simulink model "ibvs_lite_model"  (R2020b)
settings: Solver=ode45  StartTime=0.0  StopTime=inf  RelTol=1e-3  EnableMultiTasking=on
values from neighbouring files (symbols this model uses):
  q0 = zeros(7,1)    [setup.m]
  x0 = [T.t', tr2rpy(T)]    [setup.m]
undefined symbols (not defined in the file or in its folder): cond, LWR, mkgrid, nofriction, transl, troty, trotz
libraries: roblocks x19, simulink x4
(part 2 of 2)

== matlab function ibvs_lite_model/inverse_dyn ==
  data: q input; tau output; dq input; ddq input
function tau = idm(q, dq, ddq)

q1 = q(1);
q2 = q(2);
q3 = q(3);
q4 = q(4);
q5 = q(5);
q6 = q(6);
q7 = q(7);

QP1 = dq(1);
QP2 = dq(2);
QP3 = dq(3);
QP4 = dq(4);
QP5 = dq(5);
QP6 = dq(6);
QP7 = dq(7);

QDP1 = ddq(1);
QDP2 = ddq(2);
QDP3 = ddq(3);
QDP4 = ddq(4);
QDP5 = ddq(5);
QDP6 = ddq(6);
QDP7 = ddq(7);

radius = 0.05;

l1 = 0.1;
M1 = 2;

XX1 = 1/12 * M1 * l1 * l1;
XY1 = 0;
XZ1 = 0;
YY1 = 1/12 * M1 * l1 * l1;
YZ1 = 0;
ZZ1 = 1/2 * M1 * radius;
MX1 = 0;
MY1 = 0;
MZ1 = M1 * l1;

l2 = 0.1;
M2 = 2;

XX2 = 1/12 * M2 * l2 * l2;
XY2 = 0;
XZ2 = 0;
YY2 = 1/2 * M2 * radius;
YZ2 = 0;
ZZ2 = 1/12 * M2 * l2 * l2;
MX2 = 0;
MY2 = -M2 * l2;
MZ2 = 0;

l3 = 0.1;
M3 = 1.5;

XX3 = 1/12 * M3 * l3 * l3;
XY3 = 0;
XZ3 = 0;
YY3 = 1/12 * M3 * l3 * l3;
YZ3 = 0;
ZZ3 = 1/2 * M3 * radius;
MX3 = 0;
MY3 = 0;
MZ3 = M3 * l3;

l4 = 0.1;
M4 = 1.5;

XX4 = 1/12 * M4 * l4 * l4;
XY4 = 0;
XZ4 = 0;
YY4 = 1/2 * M4 * radius;
YZ4 = 0;
ZZ4 = 1/12 * M4 * l4 * l4;
MX4 = 0;
MY4 = M4 * 0.1;
MZ4 = 0;

l5 = 0.1;
M5 = 1.5;

XX5 = 1/12 * M5 * l5 * l5;
XY5 = 0;
XZ5 = 0;
YY5 = 1/12 * M5 * l5 * l5;
YZ5 = 0;
ZZ5 = 1/2 * M5 * radius;
MX5 = 0;
MY5 = 0;
MZ5 = M5 * l5;

l6 = 0.1;
M6 = 1;

XX6 = 1/12 * M6 * l6 * l6;
XY6 = 0;
XZ6 = 0;
YY6 = 1/12 * M6 * l6 * l6;
YZ6 = 0;
ZZ6 = 1/2 * M6 * radius;
MX6 = 0;
MY6 = -M6 * l6;
MZ6 = 0;

l7 = 0.05;
M7 = 0.1;

XX7 = 1/12 * M7 * l7 * l7;
XY7 = 0;
XZ7 = 0;
YY7 = 1/12 * M7 * l7 * l7;
YZ7 = 0;
ZZ7 = 1/2 * M7 * radius;
MX7 = 0;
MY7 = 0;
MZ7 = M7 * l7;


FX7 = 0;
FY7 = 0;
FZ7 = 0;
CX7 = 0;
CY7 = 0;
CZ7 = 0;
                          
C1 = cos(q1);
S1 = sin(q1);
C2 = cos(q2);
S2 = sin(q2);
C3 = cos(q3);
S3 = sin(q3);
C4 = cos(q4);
S4 = sin(q4);
C5 = cos(q5);
S5 = sin(q5);
C6 = cos(q6);
S6 = sin(q6);
C7 = cos(q7);
S7 = sin(q7);
DV61 = QP1^2;
W12 = QP1*S2;
W22 = C2*QP1;
WP12 = QDP1*S2 + QP2*W22;
WP22 = C2*QDP1 - QP2*W12;
DV12 = W12^2;
DV22 = W12*W22;
DV32 = QP2*W12;
DV42 = W22^2;
DV52 = QP2*W22;
DV62 = QP2^2;
U112 = -DV42 - DV62;
U212 = DV22 + QDP2;
U312 = DV32 - WP22;
U122 = DV22 - QDP2;
U222 = -DV12 - DV62;
U322 = DV52 + WP12;
U132 = DV32 + WP22;
U232 = DV52 - WP12;
U332 = -DV12 - DV42;
VP12 = -9.81*S2;
VP22 = -9.81*C2;
W13 = C3*W12 - QP2*S3;
W23 = -C3*QP2 - S3*W12;
W33 = QP3 + W22;
WP13 = C3*WP12 - QDP2*S3 + QP3*W23;
WP23 = -C3*QDP2 - QP3*W13 - S3*WP12;
WP33 = QDP3 + WP22;
DV13 = W13^2;
DV23 = W13*W23;
DV33 = W13*W33;
DV43 = W23^2;
DV53 = W23*W33;
DV63 = W33^2;
U113 = -DV43 - DV63;
U213 = DV23 + WP33;
U313 = DV33 - WP23;
U123 = DV23 - WP33;
U223 = -DV13 - DV63;
U323 = DV53 + WP13;
U133 = DV33 + WP23;
U233 = DV53 - WP13;
U333 = -DV13 - DV43;
VSP13 = 0.4*U112 + VP12;
VSP23 = 0.4*U212 + VP22;
VSP33 = 0.4*U312;
VP13 = C3*VSP13 - S3*VSP33;
VP23 = -C3*VSP33 - S3*VSP13;
W14 = C4*W13 - S4*W33;
W24 = -C4*W33 - S4*W13;
W34 = QP4 + W23;
WP14 = C4*WP13 + QP4*W24 - S4*WP33;
WP24 = -C4*WP33 - QP4*W14 - S4*WP13;
WP34 = QDP4 + WP23;
DV14 = W14^2;
DV24 = W14*W24;
DV34 = W14*W34;
DV44 = W24^2;
DV54 = W24*W34;
DV64 = W34^2;
U114 = -DV44 - DV64;
U214 = DV24 + WP34;
U314 = DV34 - WP24;
U124 = DV24 - WP34;
U224 = -DV14 - DV64;
U324 = DV54 + WP14;
U134 = DV34 + WP24;
U234 = DV54 - WP14;
U334 = -DV14 - DV44;
VP14 = C4*VP13 - S4*VSP23;
VP24 = -C4*VSP23 - S4*VP13;
W15 = C5*W14 + S5*W34;
W25 = C5*W34 - S5*W14;
W35 = QP5 - W24;
WP15 = C5*WP14 + QP5*W25 + S5*WP34;
WP25 = C5*WP34 - QP5*W15 - S5*WP14;
WP35 = QDP5 - WP24;
DV15 = W15^2;
DV25 = W15*W25;
DV35 = W15*W35;
DV45 = W25^2;
DV55 = W25*W35;
DV65 = W35^2;
U115 = -DV45 - DV65;
U215 = DV25 + WP35;
U315 = DV35 - WP25;
U125 = DV25 - WP35;
U225 = -DV15 - DV65;
U325 = DV55 + WP15;
U135 = DV35 + WP25;
U235 = DV55 - WP15;
U335 = -DV15 - DV45;
VSP15 = 0.39*U114 + VP14;
VSP25 = 0.39*U214 + VP24;
VSP35 = 0.39*U314 + VP23;
VP15 = C5*VSP15 + S5*VSP35;
VP25 = C5*VSP35 - S5*VSP15;
W16 = C6*W15 + S6*W35;
W26 = C6*W35 - S6*W15;
W36 = QP6 - W25;
WP16 = C6*WP15 + QP6*W26 + S6*WP35;
WP26 = C6*WP35 - QP6*W16 - S6*WP15;
WP36 = QDP6 - WP25;
DV16 = W16^2;
DV26 = W16*W26;
DV36 = W16*W36;
DV46 = W26^2;
DV56 = W26*W36;
DV66 = W36^2;
U116 = -DV46 - DV66;
U216 = DV26 + WP36;
U316 = DV36 - WP26;
U126 = DV26 - WP36;
U226 = -DV16 - DV66;
U326 = DV56 + WP16;
U136 = DV36 + WP26;
U236 = DV56 - WP16;
U336 = -DV16 - DV46;
VP16 = C6*VP15 - S6*VSP25;
VP26 = -C6*VSP25 - S6*VP15;
W17 = C7*W16 - S7*W36;
W27 = -C7*W36 - S7*W16;
W37 = QP7 + W26;
WP17 = C7*WP16 + QP7*W27 - S7*WP36;
WP27 = -C7*WP36 - QP7*W17 - S7*WP16;
WP37 = QDP7 + WP26;
DV17 = W17^2;
DV27 = W17*W27;
DV37 = W17*W37;
DV47 = W27^2;
DV57 = W27*W37;
DV67 = W37^2;
U117 = -DV47 - DV67;
U217 = DV27 + WP37;
U317 = DV37 - WP27;
U127 = DV27 - WP37;
U227 = -DV17 - DV67;
U327 = DV57 + WP17;
U137 = DV37 + WP27;
U237 = DV57 - WP17;
U337 = -DV17 - DV47;
VP17 = C7*VP16 + S7*VP25;
VP27 = C7*VP25 - S7*VP16;
F11 = -DV61*MX1 - MY1*QDP1;
F21 = -DV61*MY1 + MX1*QDP1;
F31 = -9.81*M1;
PSI11 = QP1*XZ1;
PSI21 = QP1*YZ1;
PSI31 = QP1*ZZ1;
No11 = -PSI21*QP1 + QDP1*XZ1;
No21 = PSI11*QP1 + QDP1*YZ1;
No31 = QDP1*ZZ1;
F12 = M2*VP12 + MX2*U112 + MY2*U122 + MZ2*U132;
F22 = M2*VP22 + MX2*U212 + MY2*U222 + MZ2*U232;
F32 = MX2*U312 + MY2*U322 + MZ2*U332;
PSI12 = QP2*XZ2 + W12*XX2 + W22*XY2;
PSI22 = QP2*YZ2 + W12*XY2 + W22*YY2;
PSI32 = QP2*ZZ2 + W12*XZ2 + W22*YZ2;
No12 = -PSI22*QP2 + PSI32*W22 + QDP2*XZ2 + WP12*XX2 + WP22*XY2;
No22 = PSI12*QP2 - PSI32*W12 + QDP2*YZ2 + WP12*XY2 + WP22*YY2;
No32 = -PSI12*W22 + PSI22*W12 + QDP2*ZZ2 + WP12*XZ2 + WP22*YZ2;
F13 = M3*VP13 + MX3*U113 + MY3*U123 + MZ3*U133;
F23 = M3*VP23 + MX3*U213 + MY3*U223 + MZ3*U233;
F33 = M3*VSP23 + MX3*U313 + MY3*U323 + MZ3*U333;
PSI13 = W13*XX3 + W23*XY3 + W33*XZ3;
PSI23 = W13*XY3 + W23*YY3 + W33*YZ3;
PSI33 = W13*XZ3 + W23*YZ3 + W33*ZZ3;
No13 = -PSI23*W33 + PSI33*W23 + WP13*XX3 + WP23*XY3 + WP33*XZ3;
No23 = PSI13*W33 - PSI33*W13 + WP13*XY3 + WP23*YY3 + WP33*YZ3;
No33 = -PSI13*W23 + PSI23*W13 + WP13*XZ3 + WP23*YZ3 + WP33*ZZ3;
F14 = M4*VP14 + MX4*U114 + MY4*U124 + MZ4*U134;
F24 = M4*VP24 + MX4*U214 + MY4*U224 + MZ4*U234;
F34 = M4*VP23 + MX4*U314 + MY4*U324 + MZ4*U334;
PSI14 = W14*XX4 + W24*XY4 + W34*XZ4;
PSI24 = W14*XY4 + W24*YY4 + W34*YZ4;
PSI34 = W14*XZ4 + W24*YZ4 + W34*ZZ4;
No14 = -PSI24*W34 + PSI34*W24 + WP14*XX4 + WP24*XY4 + WP34*XZ4;
No24 = PSI14*W34 - PSI34*W14 + WP14*XY4 + WP24*YY4 + WP34*YZ4;
No34 = -PSI14*W24 + PSI24*W14 + WP14*XZ4 + WP24*YZ4 + WP34*ZZ4;
F15 = M5*VP15 + MX5*U115 + MY5*U125 + MZ5*U135;
F25 = M5*VP25 + MX5*U215 + MY5*U225 + MZ5*U235;
F35 = -M5*VSP25 + MX5*U315 + MY5*U325 + MZ5*U335;
PSI15 = W15*XX5 + W25*XY5 + W35*XZ5;
PSI25 = W15*XY5 + W25*YY5 + W35*YZ5;
PSI35 = W15*XZ5 + W25*YZ5 + W35*ZZ5;
No15 = -PSI25*W35 + PSI35*W25 + WP15*XX5 + WP25*XY5 + WP35*XZ5;
No25 = PSI15*W35 - PSI35*W15 + WP15*XY5 + WP25*YY5 + WP35*YZ5;
No35 = -PSI15*W25 + PSI25*W15 + WP15*XZ5 + WP25*YZ5 + WP35*ZZ5;
F16 = M6*VP16 + MX6*U116 + MY6*U126 + MZ6*U136;
F26 = M6*VP26 + MX6*U216 + MY6*U226 + MZ6*U236;
F36 = -M6*VP25 + MX6*U316 + MY6*U326 + MZ6*U336;
PSI16 = W16*XX6 + W26*XY6 + W36*XZ6;
PSI26 = W16*XY6 + W26*YY6 + W36*YZ6;
PSI36 = W16*XZ6 + W26*YZ6 + W36*ZZ6;
No16 = -PSI26*W36 + PSI36*W26 + WP16*XX6 + WP26*XY6 + WP36*XZ6;
No26 = PSI16*W36 - PSI36*W16 + WP16*XY6 + WP26*YY6 + WP36*YZ6;
No36 = -PSI16*W26 + PSI26*W16 + WP16*XZ6 + WP26*YZ6 + WP36*ZZ6;
F17 = M7*VP17 + MX7*U117 + MY7*U127 + MZ7*U137;
F27 = M7*VP27 + MX7*U217 + MY7*U227 + MZ7*U237;
F37 = M7*VP26 + MX7*U317 + MY7*U327 + MZ7*U337;
PSI17 = W17*XX7 + W27*XY7 + W37*XZ7;
PSI27 = W17*XY7 + W27*YY7 + W37*YZ7;
PSI37 = W17*XZ7 + W27*YZ7 + W37*ZZ7;
No17 = -PSI27*W37 + PSI37*W27 + WP17*XX7 + WP27*XY7 + WP37*XZ7;
No27 = PSI17*W37 - PSI37*W17 + WP17*XY7 + WP27*YY7 + WP37*YZ7;
No37 = -PSI17*W27 + PSI27*W17 + WP17*XZ7 + WP27*YZ7 + WP37*ZZ7;
E17 = F17 + FX7;
E27 = F27 + FY7;
E37 = F37 + FZ7;
N17 = CX7 + MY7*VP26 - MZ7*VP27 + No17;
N27 = CY7 - MX7*VP26 + MZ7*VP17 + No27;
N37 = CZ7 + MX7*VP27 - MY7*VP17 + No37;
FDI17 = C7*E17 - E27*S7;
FDI37 = -C7*E27 - E17*S7;
E16 = F16 + FDI17;
E26 = E37 + F26;
E36 = F36 + FDI37;
N16 = C7*N17 - MY6*VP25 - MZ6*VP26 - N27*S7 + No16;
N26 = MX6*VP25 + MZ6*VP16 + N37 + No26;
N36 = -C7*N27 + MX6*VP26 - MY6*VP16 - N17*S7 + No36;
FDI16 = C6*E16 - E26*S6;
FDI36 = C6*E26 + E16*S6;
E15 = F15 + FDI16;
E25 = -E36 + F25;
E35 = F35 + FDI36;
N15 = C6*N16 - MY5*VSP25 - MZ5*VP25 - N26*S6 + No15;
N25 = MX5*VSP25 + MZ5*VP15 - N36 + No25;
N35 = C6*N26 + MX5*VP25 - MY5*VP15 + N16*S6 + No35;
FDI15 = C5*E15 - E25*S5;
FDI35 = C5*E25 + E15*S5;
E14 = F14 + FDI15;
E24 = -E35 + F24;
E34 = F34 + FDI35;
N14 = C5*N15 + MY4*VP23 - MZ4*VP24 - N25*S5 + No14;
N24 = -0.39*FDI35 - MX4*VP23 + MZ4*VP14 - N35 + No24;
N34 = C5*N25 - 0.39*E35 + MX4*VP24 - MY4*VP14 + N15*S5 + No34;
FDI14 = C4*E14 - E24*S4;
FDI34 = -C4*E24 - E14*S4;
E13 = F13 + FDI14;
E23 = E34 + F23;
E33 = F33 + FDI34;
N13 = C4*N14 + MY3*VSP23 - MZ3*VP23 - N24*S4 + No13;
N23 = -MX3*VSP23 + MZ3*VP13 + N34 + No23;
N33 = -C4*N24 + MX3*VP23 - MY3*VP13 - N14*S4 + No33;
FDI13 = C3*E13 - E23*S3;
FDI33 = -C3*E23 - E13*S3;
E12 = F12 + FDI13;
E22 = E33 + F22;
E32 = F32 + FDI33;
N12 = C3*N13 - MZ2*VP22 - N23*S3 + No12;
N22 = -0.4*FDI33 + MZ2*VP12 + N33 + No22;
N32 = -C3*N23 + 0.4*E33 + MX2*VP22 - MY2*VP12 - N13*S3 + No32;
FDI12 = C2*E12 - E22*S2;
FDI32 = C2*E22 + E12*S2;
E11 = F11 + FDI12;
E21 = -E32 + F21;
E31 = F31 + FDI32;
N11 = C2*N12 - 9.81*MY1 - N22*S2 + No11;
N21 = 9.81*MX1 - N32 + No21;
N31 = C2*N22 + N12*S2 + No31;
FDI11 = C1*E11 - E21*S1;
FDI21 = C1*E21 + E11*S1;
GAM1 = N31;
GAM2 = N32;
GAM3 = N33;
GAM4 = N34;
GAM5 = N35;
GAM6 = N36;
GAM7 = N37;

tau = [GAM1 GAM2 GAM3 GAM4 GAM5 GAM6 GAM7];

== matlab function ibvs_lite_model/MATLAB Function3 ==
  data: u input; y output
function y = fcn(u)

y = [0, u, 0, 0, 0, 0]';

== matlab function ibvs_lite_model/impedance ==
  data: Lambda input; f output size=6; ddx_f input; dx_f input; x_f input; x input; dx input
function f = fcn(Lambda, ddx_f, dx_f, x_f, x, dx)

M = 6;

Mv = 1 * eye(M, M);
Kd = 10 * eye(M, M);
Kp = 10 * eye(M, M);

Lambda = eye(M, M);
f = Lambda * (ddx_f + inv(Mv) * (Kd * (dx_f - dx) + Kp * (x_f - x)));
